simulink model "bat"  (R2026a)
settings: Solver=VariableStepAuto
libraries: fl_lib x2, nesl_utility x2

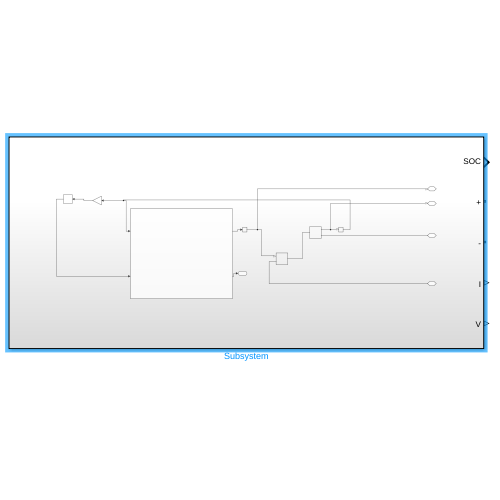
[thumbnail: Simulink's stored preview of the top-level diagram]
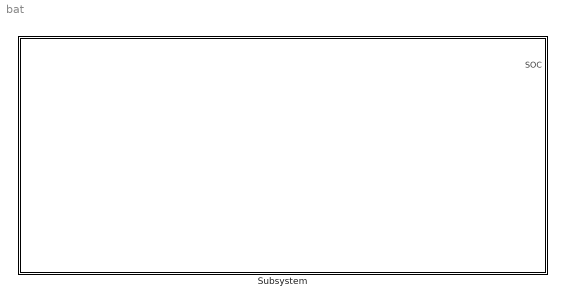
== system bat ==
  Subsystem : Subsystem

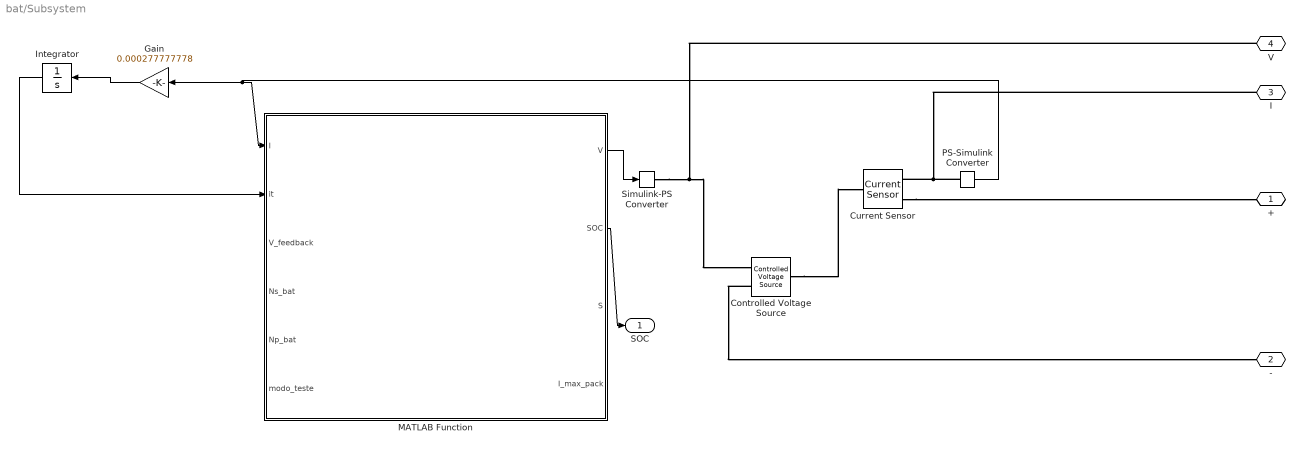
== system bat/Subsystem ==
  Controlled Voltage Source : fl_lib/Electrical/Electrical Sources/Controlled Voltage Source
  Current Sensor : fl_lib/Electrical/Electrical Sensors/Current Sensor
  Gain : Gain  Gain=0.000277777778
  Integrator : Integrator
  MATLAB Function : MATLAB Function  TreatAsAtomicUnit=on
  PS-Simulink Converter : nesl_utility/PS-Simulink Converter  PhysicalDomain=network_engine_domain  SubClassName=ps_output  LeftPortType=input  RightPortType=output  PseudoPeriodic=off  Frequencies=[]  VectorFormat=inherit  Unit=inherit  AffineConversion=off
  Simulink-PS Converter : nesl_utility/Simulink-PS Converter  PhysicalDomain=network_engine_domain  SubClassName=ps_input  LeftPortType=input  RightPortType=output  PseudoPeriodic=off  Frequencies=[]  NoiseDistribution=none  NoiseParameters=[]  Unit=1  AffineConversion=off  FilteringAndDerivatives=provide  SimscapeFilterOrder=1  InputFilterTimeConstant=0.001  UdotUserProvided=0
  + : PMIOPort  Side=Right
  - : PMIOPort  Port=2  Side=Right
  I : PMIOPort  Port=3  Side=Right
  V : PMIOPort  Port=4  Side=Right
  SOC : Outport
  wires:
  Gain/1 -> Integrator/1
  MATLAB Function/2(SOC) -> SOC/1
  MATLAB Function/1(V) -> Simulink-PS Converter/1
  Integrator/1 -> MATLAB Function/2(it)
  PS-Simulink Converter/1 -> Gain/1, MATLAB Function/1(I)
  connections:
  Controlled Voltage Source/RConn2 -- -/RConn1
  PS-Simulink Converter/LConn1 -- I/RConn1 -- Current Sensor/RConn1
  Simulink-PS Converter/RConn1 -- V/RConn1 -- Controlled Voltage Source/RConn1
  Current Sensor/RConn2 -- +/RConn1
  Controlled Voltage Source/LConn1 -- Current Sensor/LConn1

== matlab function bat/Subsystem/MATLAB Function ==
  data: I input; V output; it input; SOC output; V_feedback input; Ns_bat input; Np_bat input; modo_teste input; S output; I_max_pack output
function [V, SOC, S,I_max_pack] = modelo_bateria(I, it, V_feedback, Ns_bat, Np_bat, modo_teste)
    % ---- JH Power LiFePO4 12.8V 15Ah (4S) ----
    E0_1 = 13.32;      % constante do modelo Tremblay-Dessaint (estimado, sem curva real)
    Q_1_real  = 15;    % capacidade nominal - CONFIRMADO (15Ah / 192Wh)
    R_1  = 0.025;      % resistencia interna - ESTIMADO (sem datasheet)
    K_1_real  = 0.0444; % ESTIMADO
    A_1  = 1.4;         % ESTIMADO
    B_1_real  = 6.0;    % ESTIMADO
    V_max_1 = 14.6;    % tensao de carga - CONFIRMADO (escrito na bateria: 14.4~14.6V)
    V_min_1 = 10.0;    % corte minimo - estimado (padrao de mercado, nao veio na bateria)
    margem_religa_1 = 0.3;
    C = 15;            % 1C = 15A
    I_max_desc = 30;   % CONFIRMADO (descarga max, escrito na bateria)
    I_max_carga = 15;  % CONFIRMADO (carga max do BMS, escrito na bateria)
    % ---- Modo teste: encolhe Q (e escala K, B pelo mesmo fator) ----
    % para ver a curva de carga/descarga em segundos em vez de horas.
    % A NÃO escala. NUNCA usar modo_teste=1 para resultado final.
    if modo_teste == 1
        Q_1 = 0.00055;
        f = Q_1_real / Q_1;
        K_1 = K_1_real * f;
        B_1 = B_1_real * f;
    else
        Q_1 = Q_1_real;
        K_1 = K_1_real;
        B_1 = B_1_real;
    end

    % ---- Escala pro banco (Ns_bat em série, Np_bat em paralelo) ----
    E0 = E0_1 * Ns_bat;
    Q  = Q_1  * Np_bat;
    R  = R_1  * Ns_bat / Np_bat;
    K  = K_1  * Ns_bat;
    A  = A_1  * Ns_bat;
    B  = B_1  / Np_bat;
    V_max = V_max_1 * Ns_bat;
    V_min = V_min_1 * Ns_bat;
    margem_religa = margem_religa_1 * Ns_bat;

    if I < 0
        I_max_pack = I_max_carga * Np_bat;
    else
        I_max_pack = I_max_desc * Np_bat;
    end

    it_c = min(max(it, 0), 0.99*Q);
    E = E0 - K*(Q/(Q - it_c))*it_c + A*exp(-B*it_c);
    V = E - I*R;
    SOC = 100*(1 - it/Q);
    if SOC < 0
        SOC = 0;
    elseif SOC > 100
        SOC = 100;
    end
    % --- Lógica de proteção/religamento ---
    if V < V_min || SOC <= 0
        if V_feedback > (E + margem_religa)
            S = 1;
        else
            S = 0;
        end
    elseif V > V_max
        S = 0;
    elseif SOC >= 100 && I < 0
        S = 0;   % bloqueia carga quando já está cheia
    else
        S = 1;
    end
    if V < V_min
        V = V_min;
    elseif V > V_max
        V = V_max;
    end
end
